simulink model "Rider_PI"  (R2014b)
settings: Solver=ode45  StartTime=0.0  StopTime=10.0  RelTol=1e-3
model workspace: external: MAT-File Rider_PI.mat (data not in the file)
values from neighbouring files (symbols this model uses):
  Rider_I = Simulink.Parameter    [Pikes_Peak_generate_parameters.m]    (also in RW3_generate_parameters.m)
  Rider_P = Simulink.Parameter    [Pikes_Peak_generate_parameters.m]    (also in RW3_generate_parameters.m)
  SpeedProfile_x = Simulink.Parameter    [Pikes_Peak_generate_parameters.m]    (also in RW3_generate_parameters.m)
  SpeedProfile_y = Simulink.Parameter    [Pikes_Peak_generate_parameters.m]    (also in RW3_generate_parameters.m)
libraries: simulink x1
settings Model: Creator=Nathan  LastModifiedBy=Nathan
settings DebuggingCC: UnderspecifiedInitializationDetection=Classic  MergeDetectMultiDrivingBlocksExec=none  StateNameClashWarn=warning

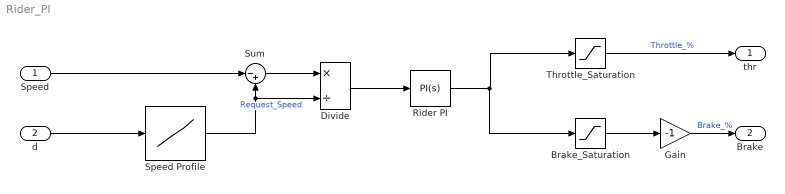
== system Rider_PI ==
  Speed : Inport
  d : Inport  Port=2
  Brake_Saturation : Saturate  UpperLimit=0  LowerLimit=-1  ZeroCross=off
  Divide : Product  Inputs=*/
  Gain : Gain  Gain=-1
  Rider PI : simulink/Continuous/PID Controller  Controller=PI  TimeDomain=Continuous-time  SampleTime=-1  IntegratorMethod=Forward Euler  FilterMethod=Forward Euler  Form=Parallel  P=Rider_P  I=Rider_I  D=0  N=100  InitialConditionSource=internal  InitialConditionForIntegrator=0  InitialConditionForFilter=0  ExternalReset=none  ZeroCross=off  LimitOutput=off  UpperSaturationLimit=inf  LowerSaturationLimit=-inf  LinearizeAsGain=on  AntiWindupMode=none  Kb=1  TrackingMode=off  Kt=1  PParamMin=[]  PParamMax=[]  IParamMin=[]  IParamMax=[]  DParamMin=[]  DParamMax=[]  NParamMin=[]  NParamMax=[]  KbParamMin=[]  KbParamMax=[]  KtParamMin=[]  KtParamMax=[]  POutMin=[]  POutMax=[]  IOutMin=[]  IOutMax=[]  DOutMin=[]  DOutMax=[]  NOutMin=[]  NOutMax=[]  KbOutMin=[]  KbOutMax=[]  KtOutMin=[]  KtOutMax=[]  IntegratorOutMin=[]  IntegratorOutMax=[]  FilterOutMin=[]  FilterOutMax=[]  SumOutMin=[]  SumOutMax=[]  SumI1OutMin=[]  SumI1OutMax=[]  SumI2OutMin=[]  SumI2OutMax=[]  SumI3OutMin=[]  SumI3OutMax=[]  SumDOutMin=[]  SumDOutMax=[]  SaturationOutMin=[]  SaturationOutMax=[]  IntegratorContinuousStateAttributes=''  IntegratorStateMustResolveToSignalObject=off  IntegratorRTWStateStorageClass=Auto  FilterContinuousStateAttributes=''  FilterStateMustResolveToSignalObject=off  FilterRTWStateStorageClass=Auto  DifferentiatorICPrevScaledInput=0  DifferentiatorOutMin=[]  DifferentiatorOutMax=[]  UseFilter=on
  Speed Profile : Lookup_n-D  NumberOfTableDimensions=1  BreakpointsForDimension1=SpeedProfile_x  Table=SpeedProfile_y  InternalRulePriority=Speed  RndMeth=Simplest  InputSameDT=on
  Sum : Sum  Inputs=|-+
  Throttle_Saturation : Saturate  UpperLimit=1  LowerLimit=0  ZeroCross=off
  thr : Outport
  Brake : Outport  Port=2
  wires:
  Speed/1 -> Sum/1
  Speed Profile/1 -> Divide/2, Sum/2  "Request_Speed"
  Sum/1 -> Divide/1
  Divide/1 -> Rider PI/1
  Throttle_Saturation/1 -> thr/1  "Throttle_%"
  Rider PI/1 -> Brake_Saturation/1, Throttle_Saturation/1
  Brake_Saturation/1 -> Gain/1
  Gain/1 -> Brake/1  "Brake_%"
  d/1 -> Speed Profile/1
